simulink model "sampleModel1436"  (R2023a)
settings: Solver=VariableStepAuto  StartTime=0.0  StopTime=10.0  RelTol=1e-3
libraries: hdlsllib x8, simulink x4
settings Model: Creator=user1  LastModifiedBy=user1

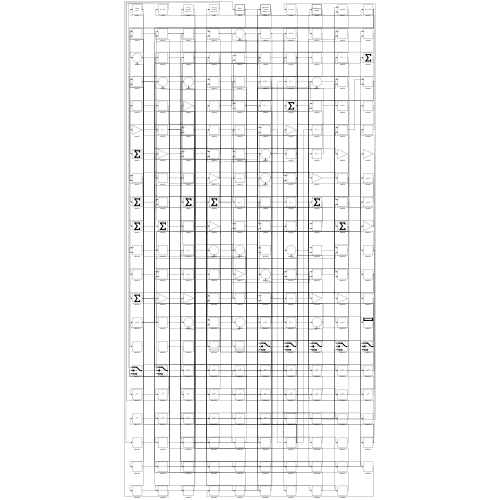
[thumbnail: Simulink's stored preview of the top-level diagram]
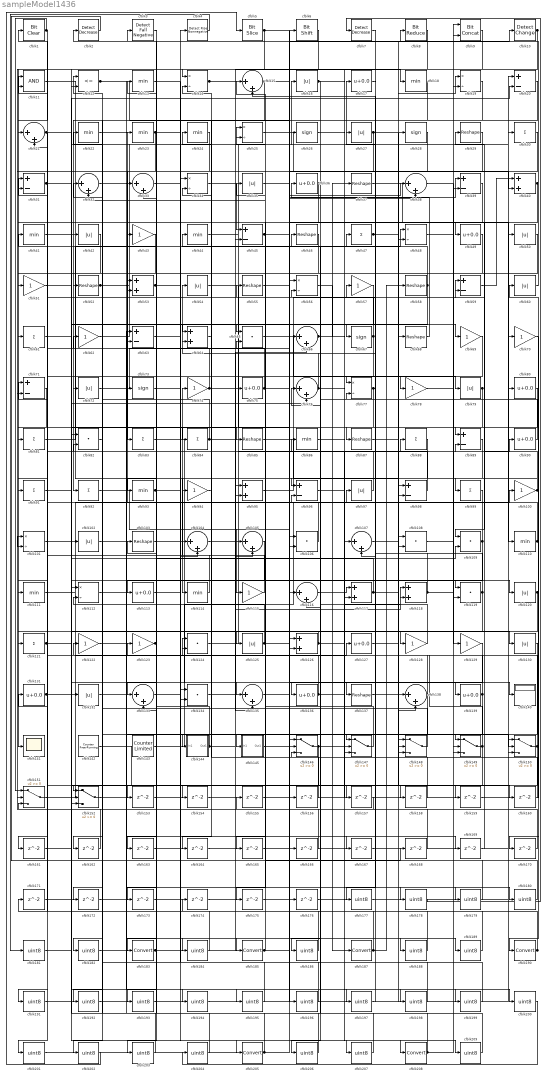
== system sampleModel1436 ==
  cfblk1 : simulink/Logic and Bit Operations/Bit Clear  iBit=0
      settings: LibrarySourceBlock=|
      | hdlsllib/Logic and Bit
      | Operations/Bit Clear
  cfblk10 : simulink/Logic and Bit Operations/Detect Change  vinit=0  OutDataTypeStr=boolean
      settings: LibrarySourceBlock=|
      | hdlsllib/Logic and Bit
      | Operations/Detect
      | Change
  cfblk{43,51,57,62,69..70,74,78,94,100,115,122..123,128..129} (15 alike) : Gain
  cfblk{14,19,25,34,48,56,77,101,112} (9 alike) : Product  Inputs=*/  RndMeth=Zero  SaturateOnIntegerOverflow=on
  cfblk{16,27,35,42,50,54,60,72,79,97,102,120,125,130,132} (15 alike) : Abs  SaturateOnIntegerOverflow=off
  cfblk{29,37,46,52,55,58,68,85,87,103,137} (11 alike) : Reshape
  cfblk{15,21,32..33,38,66,76,104..105,107,116,133,135,138} (14 alike) : Sum  Inputs=|++
  cfblk{65,82,106,108..109,119,124,134} (8 alike) : DotProduct  OutDataTypeStr=Inherit: Inherit via internal rule
  cfblk11 : Logic  AllPortsSameDT=off  OutDataTypeStr=boolean
  cfblk{13,18,22..24,41,44,86,93,110..111,114} (12 alike) : MinMax
  cfblk{17,36,49,75,80,90,113,127,131,136,139} (11 alike) : Bias  Bias=0.0  SaturateOnIntegerOverflow=off
  cfblk{40,53,64,95,117..118,126} (7 alike) : Sum
  cfblk12 : RelationalOperator  Operator=<=  OutDataTypeStr=boolean  InputSameDT=off
  cfblk{30,47,61,81,83..84,88,91..92,99,121} (11 alike) : Sum  Inputs=+
  cfblk140 : Display
  cfblk141 : Scope
  cfblk142 : hdlsllib/Sources/Counter Free-Running  NumBits=16  tsamp=-1
  cfblk143 : hdlsllib/Sources/Counter Limited  uplimit=7  tsamp=-1
  cfblk144 : Subsystem
      settings: LibrarySourceBlock=|
      | hdlsllib/Ports &
      | Subsystems/Subsystem
  cfblk145 : Subsystem
      settings: LibrarySourceBlock=|
      | hdlsllib/Ports &
      | Subsystems/Subsystem
  cfblk{146..152} (7 alike) : Switch  SaturateOnIntegerOverflow=off  InputSameDT=off
  cfblk{153..176} (24 alike) : Delay  SampleTime=1
  cfblk{177..182,184,186,188..189,191..204,206..207,209} (27 alike) : DataTypeConversion  OutDataTypeStr=uint8  SaturateOnIntegerOverflow=off  RndMeth=Floor
  cfblk{183,185,187,190,205,208} (6 alike) : DataTypeConversion  SaturateOnIntegerOverflow=off  RndMeth=Floor
  cfblk2 : simulink/Logic and Bit Operations/Detect Decrease  vinit=0.0  OutDataTypeStr=boolean
      settings: LibrarySourceBlock=|
      | hdlsllib/Logic and Bit
      | Operations/Detect
      | Decrease
  cfblk{20,31,39,45,59,63,71,89,96,98} (10 alike) : Sum  Inputs=+-
  cfblk{26,28,67,73} (4 alike) : Signum
  cfblk3 : hdlsllib/Logic and Bit Operations/Detect Fall Negative  vinit=0  OutDataTypeStr=boolean
  cfblk4 : hdlsllib/Logic and Bit Operations/Detect Rise Nonnegative  vinit=0  OutDataTypeStr=boolean
  cfblk5 : hdlsllib/Logic and Bit Operations/Bit Slice  lidx=7  ridx=0
  cfblk6 : hdlsllib/Logic and Bit Operations/Bit Shift  mode=Shift Left Logical  N=0
  cfblk7 : simulink/Logic and Bit Operations/Detect Decrease  vinit=0.0  OutDataTypeStr=boolean
      settings: LibrarySourceBlock=|
      | hdlsllib/Logic and Bit
      | Operations/Detect
      | Decrease
  cfblk8 : hdlsllib/Logic and Bit Operations/Bit Reduce  mode=AND
  cfblk9 : hdlsllib/Logic and Bit Operations/Bit Concat  numInputs=2
  wires:
  cfblk81/1 -> cfblk48/1
  cfblk124/1 -> cfblk90/1
  cfblk106/1 -> cfblk23/1
  cfblk65/1 -> cfblk79/1
  cfblk152/1 -> cfblk60/1
  cfblk83/1 -> cfblk135/1
  cfblk68/1 -> cfblk36/1
  cfblk151/1 -> cfblk127/1
  cfblk56/1 -> cfblk187/1
  cfblk20/1 -> cfblk92/1
  cfblk59/1 -> cfblk40/1
  cfblk11/1 -> cfblk114/1
  cfblk114/1 -> cfblk74/1
  cfblk128/1 -> cfblk46/1
  cfblk88/1 -> cfblk94/1
  cfblk48/1 -> cfblk129/1
  cfblk12/1 -> cfblk126/1, cfblk180/1
  cfblk120/1 -> cfblk145/1(In1), cfblk186/1
  cfblk52/1 -> cfblk17/1, cfblk69/1, cfblk184/1
  cfblk29/1 -> cfblk83/1
  cfblk131/1 -> cfblk28/1, cfblk140/1, cfblk76/2
  cfblk75/1 -> cfblk54/1, cfblk38/2
  cfblk26/1 -> cfblk78/1
  cfblk95/1 -> cfblk59/1
  cfblk103/1 -> cfblk185/1
  cfblk62/1 -> cfblk25/1
  cfblk111/1 -> cfblk119/1
  cfblk42/1 -> cfblk52/1
  cfblk71/1 -> cfblk141/1
  cfblk60/1 -> cfblk2/1
  cfblk5/1 -> cfblk14/1, cfblk40/2
  cfblk126/1 -> cfblk121/1, cfblk89/2, cfblk118/2
  cfblk101/1 -> cfblk30/1
  cfblk35/1 -> cfblk66/1
  cfblk63/1 -> cfblk205/1
  cfblk36/1 -> cfblk164/1, cfblk165/1
  cfblk41/1 -> cfblk102/1
  cfblk6/1 -> cfblk81/1
  cfblk97/1 -> cfblk22/1
  cfblk44/1 -> cfblk16/1
  cfblk18/1 -> cfblk67/1
  cfblk23/1 -> cfblk104/2, cfblk191/1
  cfblk28/1 -> cfblk96/1
  cfblk85/1 -> cfblk98/2
  cfblk64/1 -> cfblk24/1
  cfblk79/1 -> cfblk89/1, cfblk161/1
  cfblk40/1 -> cfblk61/1, cfblk109/1
  cfblk148/1 -> cfblk62/1
  cfblk91/1 -> cfblk132/1
  cfblk19/1 -> cfblk84/1
  cfblk17/1 -> cfblk107/2
  cfblk66/1 -> cfblk37/1, cfblk169/1
  cfblk143/1 -> cfblk9/1
  cfblk21/1 -> cfblk91/1, cfblk65/1
  cfblk104/1 -> cfblk20/1
  cfblk27/1 -> cfblk149/1, cfblk45/2
  cfblk96/1 -> cfblk139/1
  cfblk87/1 -> cfblk148/2
  cfblk90/1 -> cfblk44/1
  cfblk31/1 -> cfblk26/1, cfblk117/2, cfblk154/1
  cfblk146/1 -> cfblk182/1, cfblk189/1
  cfblk99/1 -> cfblk96/2
  cfblk22/1 -> cfblk128/1
  cfblk94/1 -> cfblk144/1(In1)
  cfblk34/1 -> cfblk45/1
  cfblk25/1 -> cfblk138/1
  cfblk125/1 -> cfblk32/1, cfblk38/1
  cfblk1/1 -> cfblk151/1, cfblk21/1
  cfblk92/1 -> cfblk115/1
  cfblk46/1 -> cfblk72/1
  cfblk38/1 -> cfblk119/2
  cfblk15/1 -> cfblk49/1, cfblk152/1
  cfblk47/1 -> cfblk108/1, cfblk87/1
  cfblk149/1 -> cfblk124/1, cfblk201/1
  cfblk78/1 -> cfblk120/1
  cfblk58/1 -> cfblk15/1, cfblk152/3
  cfblk16/1 -> cfblk136/1, cfblk130/1
  cfblk119/1 -> cfblk15/2, cfblk173/1
  cfblk45/1 -> cfblk6/1, cfblk147/3
  cfblk129/1 -> cfblk146/2
  cfblk117/1 -> cfblk148/3, cfblk73/1
  cfblk80/1 -> cfblk134/2
  cfblk86/1 -> cfblk208/1
  cfblk116/1 -> cfblk117/1
  cfblk105/1 -> cfblk113/1
  cfblk14/1 -> cfblk105/1, cfblk18/1
  cfblk77/1 -> cfblk57/1, cfblk162/1
  cfblk61/1 -> cfblk85/1
  cfblk32/1 -> cfblk64/1
  cfblk37/1 -> cfblk110/1
  cfblk84/1 -> cfblk95/1, cfblk66/2, cfblk12/1
  cfblk138/1 -> cfblk123/1, cfblk157/1
  cfblk147/1 -> cfblk32/2
  cfblk134/1 -> cfblk137/1
  cfblk70/1 -> cfblk190/1
  cfblk49/1 -> cfblk147/1
  cfblk144/1(Out1) -> cfblk41/1, cfblk118/1
  cfblk139/1 -> cfblk65/2, cfblk172/1
  cfblk51/1 -> cfblk20/2
  cfblk115/1 -> cfblk11/1
  cfblk54/1 -> cfblk126/2
  cfblk136/1 -> cfblk88/1, cfblk116/2, cfblk112/2
  cfblk39/1 -> cfblk93/1
  cfblk67/1 -> cfblk31/1, cfblk111/1
  cfblk107/1 -> cfblk19/1
  cfblk53/1 -> cfblk104/1, cfblk193/1
  cfblk145/1(Out1) -> cfblk8/1
  cfblk9/1 -> cfblk101/2
  cfblk76/1 -> cfblk35/1, cfblk178/1
  cfblk110/1 -> cfblk47/1, cfblk170/1
  cfblk30/1 -> cfblk77/1
  cfblk10/1 -> cfblk152/2, cfblk12/2, cfblk203/1
  cfblk109/1 -> cfblk133/1, cfblk11/2
  cfblk108/1 -> cfblk9/2
  cfblk74/1 -> cfblk135/2, cfblk13/1, cfblk21/2
  cfblk150/1 -> cfblk71/1, cfblk34/2, cfblk153/1
  cfblk123/1 -> cfblk53/1, cfblk133/2
  cfblk118/1 -> cfblk100/1, cfblk64/2
  cfblk72/1 -> cfblk39/1
  cfblk100/1 -> cfblk29/1, cfblk99/1
  cfblk102/1 -> cfblk150/2
  cfblk93/1 -> cfblk106/2, cfblk138/2
  cfblk89/1 -> cfblk108/2
  cfblk127/1 -> cfblk10/1
  cfblk121/1 -> cfblk125/1, cfblk109/2, cfblk209/1
  cfblk24/1 -> cfblk71/2
  cfblk8/1 -> cfblk147/2
  cfblk3/1 -> cfblk183/1
  cfblk98/1 -> cfblk31/2
  cfblk50/1 -> cfblk51/1
  cfblk153/1 -> cfblk105/2
  cfblk154/1 -> cfblk48/2
  cfblk155/1 -> cfblk107/1
  cfblk156/1 -> cfblk124/2
  cfblk157/1 -> cfblk151/3
  cfblk135/1 -> cfblk158/1
  cfblk158/1 -> cfblk14/2
  cfblk13/1 -> cfblk159/1
  cfblk159/1 -> cfblk150/1
  cfblk137/1 -> cfblk160/1
  cfblk160/1 -> cfblk25/2
  cfblk162/1 -> cfblk101/1
  cfblk57/1 -> cfblk163/1
  cfblk163/1 -> cfblk146/1
  cfblk164/1 -> cfblk148/1
  cfblk165/1 -> cfblk150/3
  cfblk166/1 -> cfblk1/1
  cfblk112/1 -> cfblk167/1
  cfblk167/1 -> cfblk98/1
  cfblk2/1 -> cfblk168/1
  cfblk168/1 -> cfblk151/2
  cfblk169/1 -> cfblk59/2
  cfblk170/1 -> cfblk146/3
  cfblk171/1 -> cfblk19/2
  cfblk172/1 -> cfblk95/2
  cfblk173/1 -> cfblk34/1
  cfblk174/1 -> cfblk149/2
  cfblk69/1 -> cfblk175/1
  cfblk175/1 -> cfblk149/3
  cfblk7/1 -> cfblk177/1
  cfblk177/1 -> cfblk50/1
  cfblk178/1 -> cfblk7/1
  cfblk55/1 -> cfblk179/1
  cfblk179/1 -> cfblk97/1
  cfblk180/1 -> cfblk55/1
  cfblk4/1 -> cfblk181/1
  cfblk181/1 -> cfblk42/1
  cfblk182/1 -> cfblk4/1
  cfblk183/1 -> cfblk75/1, cfblk116/1
  cfblk184/1 -> cfblk3/1
  cfblk185/1 -> cfblk156/1, cfblk155/1
  cfblk186/1 -> cfblk103/1
  cfblk187/1 -> cfblk171/1, cfblk53/2, cfblk131/1, cfblk76/1, cfblk58/1
  cfblk73/1 -> cfblk188/1
  cfblk188/1 -> cfblk56/1
  cfblk189/1 -> cfblk56/2
  cfblk190/1 -> cfblk174/1, cfblk77/2
  cfblk191/1 -> cfblk70/1
  cfblk43/1 -> cfblk192/1
  cfblk192/1 -> cfblk68/1
  cfblk193/1 -> cfblk43/1
  cfblk122/1 -> cfblk194/1
  cfblk194/1 -> cfblk80/1
  cfblk132/1 -> cfblk195/1
  cfblk195/1 -> cfblk122/1
  cfblk142/1 -> cfblk196/1
  cfblk196/1 -> cfblk134/1
  cfblk33/1 -> cfblk197/1
  cfblk197/1 -> cfblk27/1
  cfblk161/1 -> cfblk198/1
  cfblk198/1 -> cfblk33/1
  cfblk113/1 -> cfblk199/1
  cfblk199/1 -> cfblk33/2
  cfblk176/1 -> cfblk200/1
  cfblk201/1 -> cfblk176/1
  cfblk82/1 -> cfblk202/1
  cfblk202/1 -> cfblk5/1
  cfblk203/1 -> cfblk82/1
  cfblk200/1 -> cfblk204/1
  cfblk204/1 -> cfblk82/2
  cfblk205/1 -> cfblk166/1, cfblk112/1
  cfblk130/1 -> cfblk206/1
  cfblk206/1 -> cfblk63/1
  cfblk133/1 -> cfblk207/1
  cfblk207/1 -> cfblk63/2
  cfblk208/1 -> cfblk39/2, cfblk106/1
  cfblk209/1 -> cfblk86/1

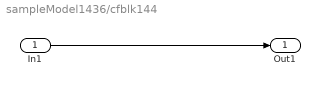
== system sampleModel1436/cfblk144 ==
  In1 : Inport
  Out1 : Outport
  wires:
  In1/1 -> Out1/1

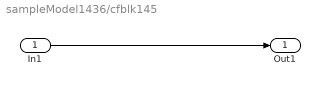
== system sampleModel1436/cfblk145 ==
  In1 : Inport
  Out1 : Outport
  wires:
  In1/1 -> Out1/1
